simulink model "QAM64"  (R2017a)
settings: Solver=VariableStepAuto  StartTime=0.0  StopTime=9600*Tb  RelTol=1e-3
values from neighbouring files (symbols this model uses):
  Tb = 5e-8    (= 5e-08)    [cuatrobits.m]    (also in dosbits.m; seisbits.m; tresbits.m)
libraries: commfilt2 x4, commdigbbndam3 x2, dspsigops x2, simulink x1
settings Model: Creator=se.alfonso  LastModifiedBy=se.alfonso

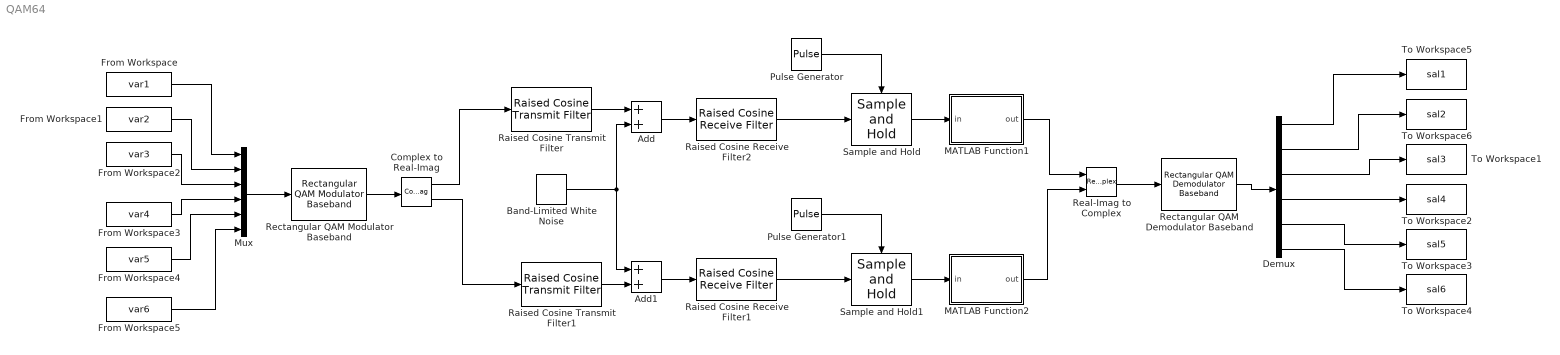
== system QAM64 ==
  Add : Sum
  Add1 : Sum
  Band-Limited White Noise : simulink/Sources/Band-Limited White Noise  Cov=No  Ts=Tb  seed=[23341]
  Complex to Real-Imag : ComplexToRealImag
  Demux : Demux  Outputs=6
  From Workspace : FromWorkspace  VariableName=var1  SampleTime=Tb
  From Workspace1 : FromWorkspace  VariableName=var2  SampleTime=Tb
  From Workspace2 : FromWorkspace  VariableName=var3  SampleTime=Tb
  From Workspace3 : FromWorkspace  VariableName=var4  SampleTime=Tb
  From Workspace4 : FromWorkspace  VariableName=var5  SampleTime=Tb
  From Workspace5 : FromWorkspace  VariableName=var6  SampleTime=Tb
  MATLAB Function1 : MATLAB Function  TreatAsAtomicUnit=on
  MATLAB Function2 : MATLAB Function  TreatAsAtomicUnit=on
  Mux : Mux  Inputs=6
  Pulse Generator : DiscretePulseGenerator  PulseType=Time based  Period=6*Tb  PulseWidth=50
  Pulse Generator1 : DiscretePulseGenerator  PulseType=Time based  Period=6*Tb  PulseWidth=50
  Raised Cosine Receive Filter1 : commfilt2/Raised Cosine Receive Filter  filtType=Square root  R=0.25  filtSpan=2  N=5  downFactor=1  downOffset=0  filterGain=1  RateOptions=Allow multirate processing  framing=Allow multirate processing  checkCoeff=off  variableName=rcRxFilt1  currentFiltSpan=2  D=(2)/2  inputOffset=0  sampMode=Mute  saveAsFlag=1  rateMode=Downsampling  checkGain=Normalized  launchFVT=on  roundingMode=Floor  overflowMode=off  coeffDataTypeStr=Inherit: Same word length as input  coeffMin=[]  coeffMax=[]  coeffLastDataTypeStr=Inherit: Same word length as input  accumDataTypeStr=Inherit: Same as product output  accumLastDataTypeStr=Inherit: Same as product output  outputDataTypeStr=Inherit: Same as accumulator  outputMin=[]  outputMax=[]  outputLastDataTypeStr=Inherit: Same as accumulator
  Raised Cosine Receive Filter2 : commfilt2/Raised Cosine Receive Filter  filtType=Square root  R=0.25  filtSpan=2  N=5  downFactor=1  downOffset=0  filterGain=1  RateOptions=Allow multirate processing  framing=Allow multirate processing  checkCoeff=off  variableName=rcRxFilt2  currentFiltSpan=2  D=(2)/2  inputOffset=0  sampMode=Mute  saveAsFlag=1  rateMode=Downsampling  checkGain=Normalized  launchFVT=on  roundingMode=Floor  overflowMode=off  coeffDataTypeStr=Inherit: Same word length as input  coeffMin=[]  coeffMax=[]  coeffLastDataTypeStr=Inherit: Same word length as input  accumDataTypeStr=Inherit: Same as product output  accumLastDataTypeStr=Inherit: Same as product output  outputDataTypeStr=Inherit: Same as accumulator  outputMin=[]  outputMax=[]  outputLastDataTypeStr=Inherit: Same as accumulator
  Raised Cosine Transmit Filter : commfilt2/Raised Cosine Transmit Filter  filtType=Square root  R=0.25  filtSpan=2  N=6  filterGain=1  RateOptions=Allow multirate processing  framing=Allow multirate processing  checkCoeff=off  variableName=rcTxFilt  checkGain=Normalized  sampMode=Mute  saveAsFlag=1  currentFiltSpan=2  D=(2)/2  launchFVT=on  roundingMode=Floor  overflowMode=off  coeffDataTypeStr=Inherit: Same word length as input  coeffMin=[]  coeffMax=[]  coeffLastDataTypeStr=Inherit: Same word length as input  outputDataTypeStr=Inherit: Same as accumulator  outputMin=[]  outputMax=[]  outputLastDataTypeStr=Inherit: Same as accumulator
  Raised Cosine Transmit Filter1 : commfilt2/Raised Cosine Transmit Filter  filtType=Square root  R=0.25  filtSpan=2  N=6  filterGain=1  RateOptions=Allow multirate processing  framing=Allow multirate processing  checkCoeff=off  variableName=rcTxFilt1  checkGain=Normalized  sampMode=Mute  saveAsFlag=1  currentFiltSpan=2  D=(2)/2  launchFVT=on  roundingMode=Floor  overflowMode=off  coeffDataTypeStr=Inherit: Same word length as input  coeffMin=[]  coeffMax=[]  coeffLastDataTypeStr=Inherit: Same word length as input  outputDataTypeStr=Inherit: Same as accumulator  outputMin=[]  outputMax=[]  outputLastDataTypeStr=Inherit: Same as accumulator
  Real-Imag to Complex : RealImagToComplex
  Rectangular QAM Demodulator Baseband : commdigbbndam3/Rectangular QAM Demodulator Baseband  M=64  OutType=Bit  DecType=Hard decision  VarSource=Dialog  Variance=1  Dec=Gray  Mapping=[0:15]  PowType=Min. distance between symbols  MinDist=200  AvgPow=1  PeakPow=1  Ph=0  outDtype1=Inherit via internal rule  outDtype2=Inherit via internal rule  derotateFactorWordLen=16  derotateFactorDataTypeStr=Inherit: Same word length as input  derotateFactorLastDataTypeStr=Inherit: Same word length as input  denormFactorWordLen=16  denormFactorDataTypeStr=Inherit: Same word length as input  denormFactorLastDataTypeStr=Inherit: Same word length as input  prodOutWordLen=32  prodOutOverflowMode=Wrap  prodOutRoundingMode=Floor  prodOutOvFlMode=off  prodOutOvFlModeLastStrValue=off  sumWordLen=32
  Rectangular QAM Modulator Baseband : commdigbbndam3/Rectangular QAM Modulator Baseband  M=64  InType=Bit  Enc=Gray  Mapping=[0:15]  PowType=Min. distance between symbols  MinDist=200  AvgPow=1  PeakPow=1  Ph=0  outDtype=double  outWordLen=16  outUDDataType=sfix(16)  outFracLenMode=Best precision  outFracLen=15  outDataTypeStr=double  outLastDataTypeStr=double
  Sample and Hold : dspsigops/Sample and Hold  trig=Rising edge  initCond=0  latchinput=off
  Sample and Hold1 : dspsigops/Sample and Hold  trig=Rising edge  initCond=0  latchinput=off
  To Workspace1 : ToWorkspace  VariableName=sal3  SampleTime=Tb
      settings: Save2DSignal=2-D array (concatenate along first dimension)
  To Workspace2 : ToWorkspace  VariableName=sal4  SampleTime=Tb
      settings: Save2DSignal=2-D array (concatenate along first dimension)
  To Workspace3 : ToWorkspace  VariableName=sal5  SampleTime=Tb
      settings: Save2DSignal=2-D array (concatenate along first dimension)
  To Workspace4 : ToWorkspace  VariableName=sal6  SampleTime=Tb
      settings: Save2DSignal=2-D array (concatenate along first dimension)
  To Workspace5 : ToWorkspace  VariableName=sal1  SampleTime=Tb
      settings: Save2DSignal=2-D array (concatenate along first dimension)
  To Workspace6 : ToWorkspace  VariableName=sal2  SampleTime=Tb
      settings: Save2DSignal=2-D array (concatenate along first dimension)
  wires:
  Real-Imag to Complex/1 -> Rectangular QAM Demodulator Baseband/1
  Pulse Generator1/1 -> Sample and Hold1/Trigger
  Raised Cosine Receive Filter2/1 -> Sample and Hold/1
  Demux/3 -> To Workspace1/1
  Complex to Real-Imag/2 -> Raised Cosine Transmit Filter1/1
  Demux/1 -> To Workspace5/1
  Demux/2 -> To Workspace6/1
  Rectangular QAM Demodulator Baseband/1 -> Demux/1
  Band-Limited White Noise/1 -> Add/2, Add1/1
  From Workspace1/1 -> Mux/2
  Complex to Real-Imag/1 -> Raised Cosine Transmit Filter/1
  Sample and Hold/1 -> MATLAB Function1/1(in)
  MATLAB Function1/1(out) -> Real-Imag to Complex/1
  Pulse Generator/1 -> Sample and Hold/Trigger
  From Workspace/1 -> Mux/1
  Rectangular QAM Modulator Baseband/1 -> Complex to Real-Imag/1
  Sample and Hold1/1 -> MATLAB Function2/1(in)
  Raised Cosine Receive Filter1/1 -> Sample and Hold1/1
  Add1/1 -> Raised Cosine Receive Filter1/1
  MATLAB Function2/1(out) -> Real-Imag to Complex/2
  Mux/1 -> Rectangular QAM Modulator Baseband/1
  Raised Cosine Transmit Filter/1 -> Add/1
  From Workspace2/1 -> Mux/3
  From Workspace3/1 -> Mux/4
  Raised Cosine Transmit Filter1/1 -> Add1/2
  Add/1 -> Raised Cosine Receive Filter2/1
  From Workspace4/1 -> Mux/5
  From Workspace5/1 -> Mux/6
  Demux/4 -> To Workspace2/1
  Demux/5 -> To Workspace3/1
  Demux/6 -> To Workspace4/1

== matlab function QAM64/MATLAB Function1 ==
  data: in input; out output
function out   = DecisionReal(in)
DisMin=200;
out=zeros(size(in),'like',in);

niv=1:8;
niv(1)=-700;
niv(2)=-500;
niv(3)=-300;
niv(4)=-100;
niv(5)=100;
niv(6)=300;
niv(7)=500;
niv(8)=700;

if in < 0
    if in < -200
        if in < -400
            if in < -600
                out=niv(1);
            end
            if in >= -600;
                out=niv(2);
            end
        end
        if in >= -400
          out=niv(3);
        end
    end
    if in >= -200
    out=niv(4);
    end
end
 
if in >= 0
    if in > 200
        if in > 400
            if in > 600
                out=niv(8);
            end
            if in <= 600;
                out=niv(7);
            end
        end
        if in <= 400
          out=niv(6);
        end
    end
    if in <= 200
    out=niv(5);
    end
end
end

== matlab function QAM64/MATLAB Function2 ==
  data: in input; out output
function out = DecisionIm(in)
DisMin=200;
out=zeros(size(in),'like',in);

niv=1:8;
niv(1)=-700;
niv(2)=-500;
niv(3)=-300;
niv(4)=-100;
niv(5)=100;
niv(6)=300;
niv(7)=500;
niv(8)=700;

if in < 0
    if in < -200
        if in < -400
            if in < -600
                out=niv(1);
            end
            if in >= -600;
                out=niv(2);
            end
        end
        if in >= -400
          out=niv(3);
        end
    end
    if in >= -200
    out=niv(4);
    end
end
 
if in >= 0
    if in > 200
        if in > 400
            if in > 600
                out=niv(8);
            end
            if in <= 600;
                out=niv(7);
            end
        end
        if in <= 400
          out=niv(6);
        end
    end
    if in <= 200
    out=niv(5);
    end
end
end
